simulink model "Quadcopter_model"  (R2022b)
settings: Solver=FixedStepAuto  StartTime=0.0  StopTime=5  FixedStep=Ts  RelTol=1e-3
undefined symbols (not defined in the file or in its folder): Cm, Ct, g, Ir, Ixx, Iyy, Izz, Length, linear_mat_A, linear_mat_B, linear_mat_C, linear_mat_D, mass
settings Model: Creator=Bw Jiang  LastModifiedBy=Bw Jiang

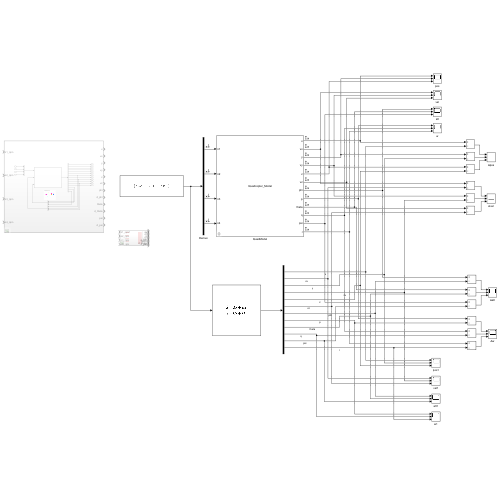
[thumbnail: Simulink's stored preview of the top-level diagram]
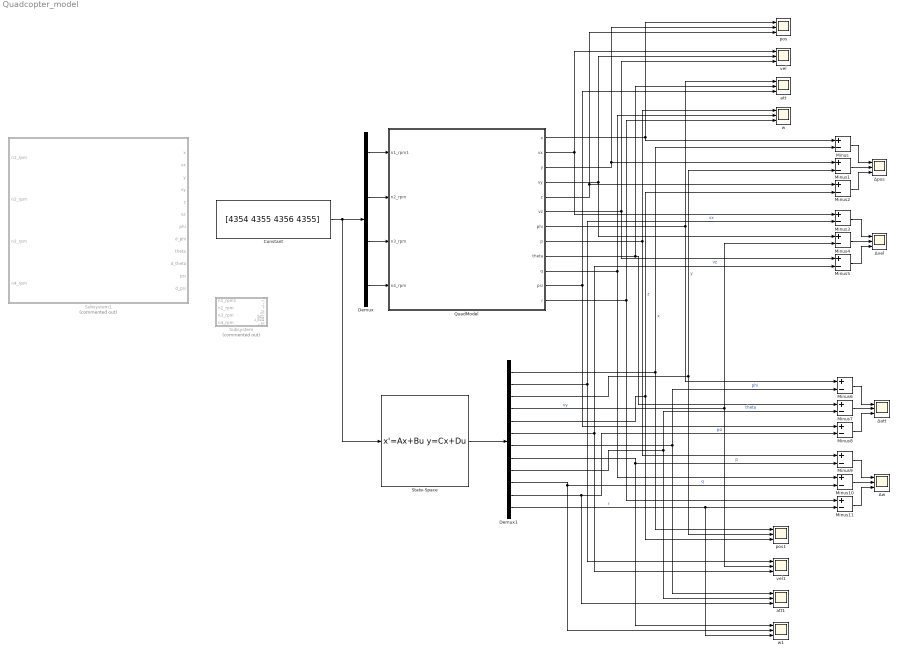
== system Quadcopter_model ==
  Constant : Constant  Value=[4354 4355 4356 4355]
  Demux : Demux
  Demux1 : Demux  Outputs=12
  Minus{,1..11} (12 alike) : Sum  Inputs=+-
  QuadModel : Subsystem  mask{g=g, mass=mass, I_xx=Ixx, I_yy=Iyy, I_zz=Izz, I_r=Ir, L=Length, C_M=Cm, C_T=Ct}
      mask prompts: g "Gravity"; I_xx "Inertia_xx"; I_yy "Inertia_yy"; I_zz "Inertia_zz"; I_r "Inertia_per_rotor"; L "Length"
      mask DialogControl ParameterGroupVar Prompt: 参数
      mask Display:
      | disp('Quadcopter_Model');
      | 
      | port_label('input', 1, 'n1');
      | port_label('input', 2, 'n2');
      | port_label('input', 3, 'n3');
      | port_label('input', 4, 'n4');
      | 
      | port_label('output', 1, 'x');
      | port_label('output', 2, 'vx');
      | port_label('output', 3, 'y');
      | port_label('output', 4, 'vy');
      | port_label('output', 5, 'z');
      | port_label('output', 6, 'vz');
      | port_label('output', 7, 'phi');
      | port_label('output', 8, 'p');
      | port_label('output', 9, 'theta');
      | port_label('output', 10, 'q');
      | port_label('output', 11, 'psi');
      | port_label('output', 12, 'r');
  State-Space : StateSpace  A=linear_mat_A  B=linear_mat_B  C=linear_mat_C  D=linear_mat_D  InitialCondition=0
  Subsystem : Subsystem  Commented=on
  Subsystem1 : Subsystem  Commented=on
  att : Scope  NumInputPorts=3
  att1 : Scope  NumInputPorts=3
  pos : Scope  NumInputPorts=3
  pos1 : Scope  NumInputPorts=3
  vel : Scope  NumInputPorts=3
  vel1 : Scope  NumInputPorts=3
  w : Scope  NumInputPorts=3
  w1 : Scope  NumInputPorts=3
  Δatt : Scope  NumInputPorts=3
  Δpos : Scope  NumInputPorts=3
  Δvel : Scope  NumInputPorts=3
  Δw : Scope  NumInputPorts=3
  wires:
  Demux/1 -> QuadModel/1(n1_rpm1)
  Demux/2 -> QuadModel/2(n2_rpm)
  Demux/3 -> QuadModel/3(n3_rpm)
  Demux/4 -> QuadModel/4(n4_rpm)
  Constant/1 -> Demux/1, State-Space/1
  QuadModel/1(x) -> Minus/1, pos/1
  QuadModel/3(y) -> pos/2, Minus1/1
  QuadModel/5(z) -> pos/3, Minus2/1
  QuadModel/2(vx) -> Minus3/1, vel/1
  QuadModel/4(vy) -> vel/2, Minus4/1
  QuadModel/6(vz) -> Minus5/1, vel/3
  QuadModel/7(phi) -> Minus6/1, att/1
  QuadModel/9(theta) -> Minus7/1, att/2
  QuadModel/11(psi) -> Minus8/1, att/3
  QuadModel/8(p) -> Minus9/1, w/1
  QuadModel/10(q) -> Minus10/1, w/2
  QuadModel/12(r) -> Minus11/1, w/3
  State-Space/1 -> Demux1/1
  Demux1/1 -> Minus/2, pos1/1  "x"
  Demux1/3 -> Minus1/2, pos1/2  "y"
  Demux1/5 -> Minus2/2, pos1/3  "z"
  Demux1/2 -> Minus3/2, vel1/1  "vx"
  Demux1/4 -> Minus4/2, vel1/2  "vy"
  Demux1/6 -> Minus5/2, vel1/3  "vz"
  Demux1/7 -> Minus6/2, att1/1  "phi"
  Demux1/9 -> Minus7/2, att1/2  "theta"
  Demux1/11 -> Minus8/2, att1/3  "psi"
  Demux1/12 -> Minus11/2, w1/3  "r"
  Demux1/10 -> w1/2, Minus10/2  "q"
  Demux1/8 -> w1/1, Minus9/2  "p"
  Minus/1 -> Δpos/1
  Minus1/1 -> Δpos/2
  Minus2/1 -> Δpos/3
  Minus3/1 -> Δvel/1
  Minus5/1 -> Δvel/3
  Minus4/1 -> Δvel/2
  Minus6/1 -> Δatt/1
  Minus7/1 -> Δatt/2
  Minus8/1 -> Δatt/3
  Minus9/1 -> Δw/1
  Minus10/1 -> Δw/2
  Minus11/1 -> Δw/3

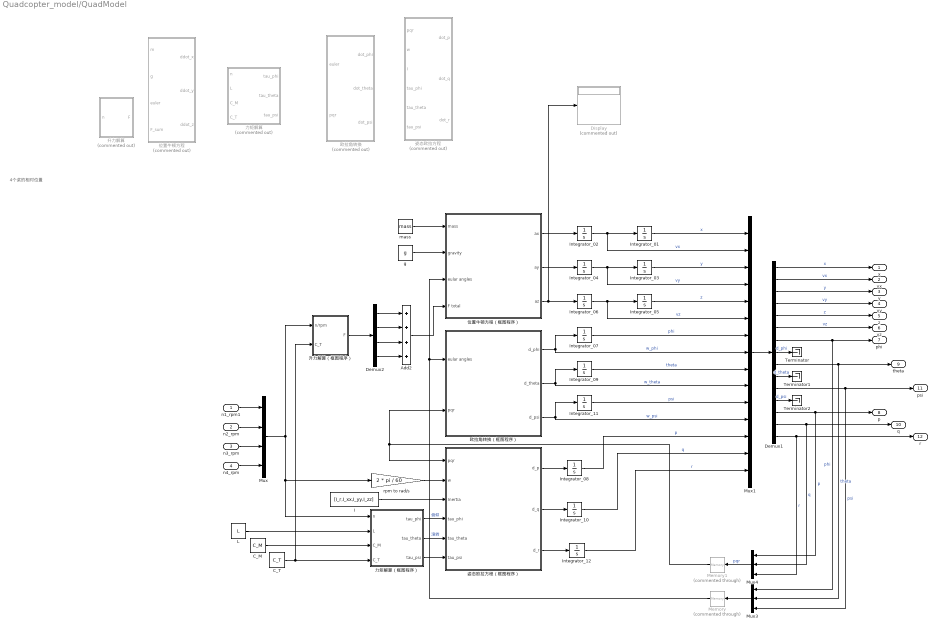
== system Quadcopter_model/QuadModel ==
  note: 4个桨的相对位置
  n1_rpm1 : Inport
  n2_rpm : Inport  Port=2
  n3_rpm : Inport  Port=3
  n4_rpm : Inport  Port=4
  Add2 : Sum  Inputs=++++
  C_M : Constant  Value=C_M
  C_T : Constant  Value=C_T
  Demux1 : Demux  Outputs=15
  Demux2 : Demux
  Display : Display  Commented=on
  I : Constant  Value=[I_r,I_xx,I_yy,I_zz]
  Integrator_01 : Integrator
  Integrator_02 : Integrator
  Integrator_03 : Integrator
  Integrator_04 : Integrator
  Integrator_05 : Integrator
  Integrator_06 : Integrator
  Integrator_07 : Integrator
  Integrator_08 : Integrator
  Integrator_09 : Integrator
  Integrator_10 : Integrator
  Integrator_11 : Integrator
  Integrator_12 : Integrator
  L : Constant  Value=L
  Memory : Memory  Commented=through  InheritSampleTime=on
  Memory1 : Memory  Commented=through  InheritSampleTime=on
  Mux : Mux
  Mux1 : Mux  Inputs=15
  Mux3 : Mux  Inputs=3
  Mux4 : Mux  Inputs=3
  Terminator : Terminator
  Terminator1 : Terminator
  Terminator2 : Terminator
  g : Constant  Value=g
  mass : Constant  Value=mass
  rpm to rad/s : Gain  Gain=2 * pi / 60
  位置牛顿方程 : MATLAB Function  Commented=on  TreatAsAtomicUnit=on
  位置牛顿方程（框图程序） : Subsystem
  力矩解算 : MATLAB Function  Commented=on  TreatAsAtomicUnit=on
  力矩解算（框图程序） : Subsystem
  升力解算 : MATLAB Function  Commented=on  TreatAsAtomicUnit=on
  升力解算（框图程序） : Subsystem
  姿态欧拉方程 : MATLAB Function  Commented=on  TreatAsAtomicUnit=on
  姿态欧拉方程（框图程序） : Subsystem
  欧拉角转换 : MATLAB Function  Commented=on  TreatAsAtomicUnit=on
  欧拉角转换（框图程序） : Subsystem
  x : Outport
  vx : Outport  Port=2
  y : Outport  Port=3
  vy : Outport  Port=4
  z : Outport  Port=5
  vz : Outport  Port=6
  phi : Outport  Port=7
  p : Outport  Port=8
  theta : Outport  Port=9
  q : Outport  Port=10
  psi : Outport  Port=11
  r : Outport  Port=12
  wires:
  Demux1/15 -> r/1, Mux4/3  "r"
  Demux1/13 -> Mux4/1, p/1  "p"
  Mux4/1 -> Memory1/1  "pqr"
  Demux1/9 -> theta/1, Mux3/2  "theta"
  Demux1/1 -> x/1  "x"
  Demux1/2 -> vx/1  "vx"
  Demux1/11 -> psi/1, Mux3/3  "psi"
  Demux1/4 -> vy/1  "vy"
  Demux1/3 -> y/1  "y"
  Demux1/5 -> z/1  "z"
  Mux1/1 -> Demux1/1
  Demux1/6 -> vz/1  "vz"
  Demux1/7 -> phi/1, Mux3/1  "phi"
  Mux3/1 -> Memory/1
  Demux1/14 -> q/1, Mux4/2  "q"
  Demux1/8 -> Terminator/1  "d_phi"
  Demux1/10 -> Terminator1/1  "d_theta"
  Demux1/12 -> Terminator2/1  "d_psi"
  n1_rpm1/1 -> Mux/1
  n2_rpm/1 -> Mux/2
  n4_rpm/1 -> Mux/4
  n3_rpm/1 -> Mux/3
  欧拉角转换（框图程序）/2(d_theta) -> Integrator_09/1, Mux1/10  "w_theta"
  欧拉角转换（框图程序）/3(d_psi) -> Integrator_11/1, Mux1/12  "w_psi"
  欧拉角转换（框图程序）/1(d_phi) -> Integrator_07/1, Mux1/8  "w_phi"
  力矩解算（框图程序）/3(tau_psi) -> 姿态欧拉方程（框图程序）/6(tau_psi)
  力矩解算（框图程序）/2(tau_theta) -> 姿态欧拉方程（框图程序）/5(tau_theta)  "滚转"
  姿态欧拉方程（框图程序）/2(d_q) -> Integrator_10/1
  姿态欧拉方程（框图程序）/3(d_r) -> Integrator_12/1
  mass/1 -> 位置牛顿方程（框图程序）/1(mass)
  Add2/1 -> 位置牛顿方程（框图程序）/4(F total)
  g/1 -> 位置牛顿方程（框图程序）/2(gravity)
  位置牛顿方程（框图程序）/3(az) -> Display/1, Integrator_06/1
  位置牛顿方程（框图程序）/2(ay) -> Integrator_04/1
  Integrator_09/1 -> Mux1/9  "theta"
  力矩解算（框图程序）/1(tau_phi) -> 姿态欧拉方程（框图程序）/4(tau_phi)  "俯仰"
  Integrator_02/1 -> Integrator_01/1, Mux1/2  "vx"
  Integrator_03/1 -> Mux1/3  "y"
  Demux2/3 -> Add2/3
  Integrator_12/1 -> Mux1/15  "r"
  rpm to rad/s/1 -> 姿态欧拉方程（框图程序）/2(w)
  Integrator_11/1 -> Mux1/11  "psi"
  Integrator_04/1 -> Mux1/4, Integrator_03/1  "vy"
  Mux/1 -> 力矩解算（框图程序）/1(n), rpm to rad/s/1, 升力解算（框图程序）/1(n/rpm)
  Memory1/1 -> 欧拉角转换（框图程序）/2(pqr), 姿态欧拉方程（框图程序）/1(pqr)
  位置牛顿方程（框图程序）/1(ax) -> Integrator_02/1
  Demux2/1 -> Add2/1
  Integrator_01/1 -> Mux1/1  "x"
  Integrator_10/1 -> Mux1/14  "q"
  姿态欧拉方程（框图程序）/1(d_p) -> Integrator_08/1
  Integrator_07/1 -> Mux1/7  "phi"
  Demux2/2 -> Add2/2
  L/1 -> 力矩解算（框图程序）/2(L)
  I/1 -> 姿态欧拉方程（框图程序）/3(Inertia)
  C_M/1 -> 力矩解算（框图程序）/3(C_M)
  升力解算（框图程序）/1(F) -> Demux2/1
  C_T/1 -> 升力解算（框图程序）/2(C_T), 力矩解算（框图程序）/4(C_T)
  Integrator_05/1 -> Mux1/5  "z"
  Demux2/4 -> Add2/4
  Integrator_06/1 -> Mux1/6, Integrator_05/1  "vz"
  Integrator_08/1 -> Mux1/13  "p"
  Memory/1 -> 位置牛顿方程（框图程序）/3(eular angles), 欧拉角转换（框图程序）/1(eular angles)

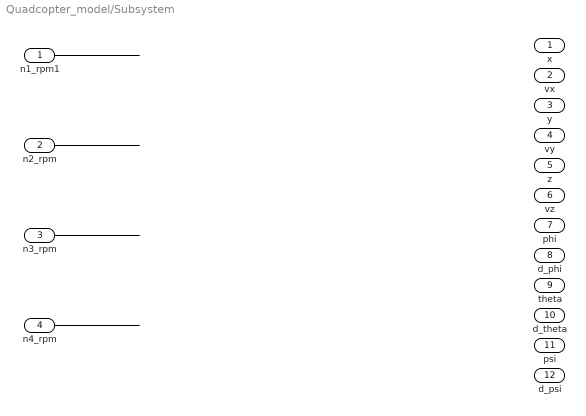
== system Quadcopter_model/Subsystem ==
  n1_rpm1 : Inport
  n2_rpm : Inport  Port=2
  n3_rpm : Inport  Port=3
  n4_rpm : Inport  Port=4
  x : Outport
  vx : Outport  Port=2
  y : Outport  Port=3
  vy : Outport  Port=4
  z : Outport  Port=5
  vz : Outport  Port=6
  phi : Outport  Port=7
  d_phi : Outport  Port=8
  theta : Outport  Port=9
  d_theta : Outport  Port=10
  psi : Outport  Port=11
  d_psi : Outport  Port=12
  wires:
  n2_rpm/1 -> ?
  n3_rpm/1 -> ?
  n4_rpm/1 -> ?
  n1_rpm1/1 -> ?
  ? -> theta/1
  ? -> x/1
  ? -> d_psi/1
  ? -> vx/1
  ? -> y/1
  ? -> vy/1
  ? -> psi/1
  ? -> d_phi/1
  ? -> vz/1
  ? -> d_theta/1
  ? -> z/1
  ? -> phi/1

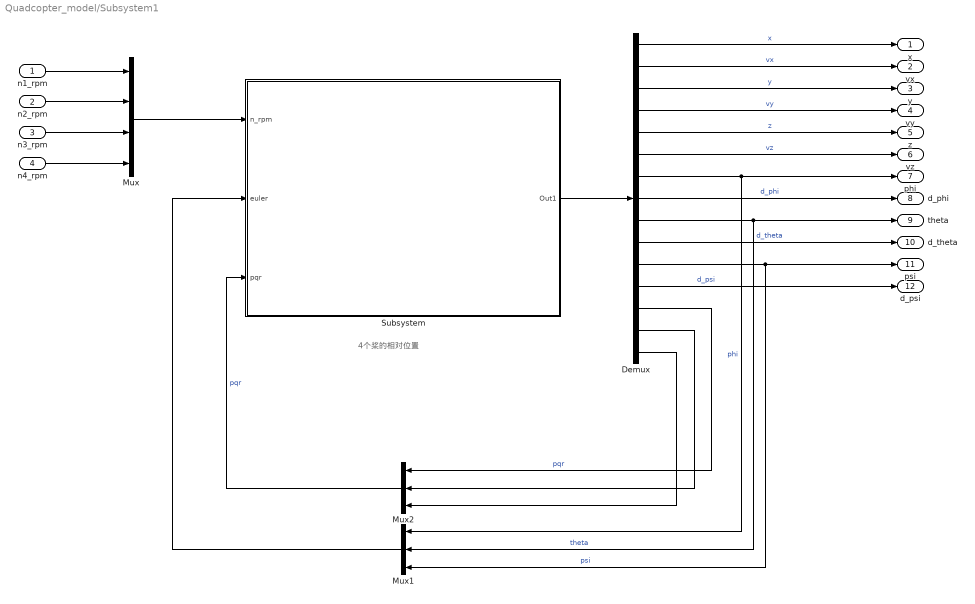
== system Quadcopter_model/Subsystem1 ==
  note: 4个桨的相对位置
  n1_rpm : Inport
  n2_rpm : Inport  Port=2
  n3_rpm : Inport  Port=3
  n4_rpm : Inport  Port=4
  Demux : Demux  Outputs=15
  Mux : Mux
  Mux1 : Mux  Inputs=3
  Mux2 : Mux  Inputs=3
  Subsystem : Subsystem
  x : Outport
  vx : Outport  Port=2
  y : Outport  Port=3
  vy : Outport  Port=4
  z : Outport  Port=5
  vz : Outport  Port=6
  phi : Outport  Port=7
  d_phi : Outport  Port=8
  theta : Outport  Port=9
  d_theta : Outport  Port=10
  psi : Outport  Port=11
  d_psi : Outport  Port=12
  wires:
  Demux/11 -> psi/1, Mux1/3  "psi"
  Demux/14 -> Mux2/2
  Mux2/1 -> Subsystem/3(pqr)  "pqr"
  Demux/13 -> Mux2/1  "pqr"
  Subsystem/1(Out1) -> Demux/1
  Demux/9 -> theta/1, Mux1/2  "theta"
  Demux/15 -> Mux2/3
  Demux/7 -> phi/1, Mux1/1  "phi"
  Demux/5 -> z/1  "z"
  Mux1/1 -> Subsystem/2(euler)
  Demux/8 -> d_phi/1  "d_phi"
  Demux/2 -> vx/1  "vx"
  n1_rpm/1 -> Mux/1
  Demux/12 -> d_psi/1  "d_psi"
  Demux/10 -> d_theta/1  "d_theta"
  Demux/4 -> vy/1  "vy"
  Demux/6 -> vz/1  "vz"
  Demux/3 -> y/1  "y"
  Demux/1 -> x/1  "x"
  n3_rpm/1 -> Mux/3
  n4_rpm/1 -> Mux/4
  n2_rpm/1 -> Mux/2
  Mux/1 -> Subsystem/1(n_rpm)

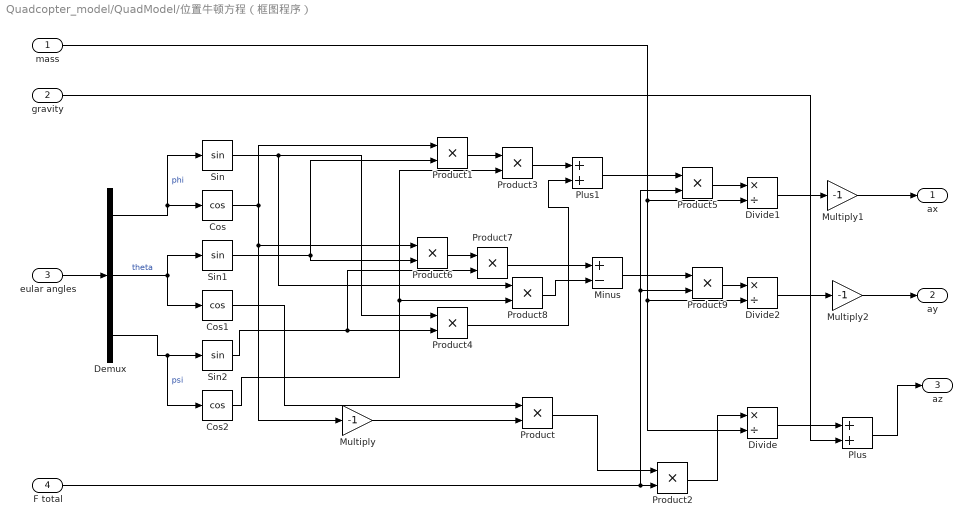
== system Quadcopter_model/QuadModel/位置牛顿方程（框图程序） ==
  mass : Inport
  gravity : Inport  Port=2
  eular angles : Inport  Port=3
  F total : Inport  Port=4
  Cos : Trigonometry  Operator=cos
  Cos1 : Trigonometry  Operator=cos
  Cos2 : Trigonometry  Operator=cos
  Demux : Demux  Outputs=3
  Divide : Product  Inputs=*/
  Divide1 : Product  Inputs=*/
  Divide2 : Product  Inputs=*/
  Minus : Sum  Inputs=+-
  Multiply : Gain  Gain=-1
  Multiply1 : Gain  Gain=-1
  Multiply2 : Gain  Gain=-1
  Plus : Sum
  Plus1 : Sum
  Product{,1..9} (10 alike) : Product
  Sin : Trigonometry
  Sin1 : Trigonometry
  Sin2 : Trigonometry
  ax : Outport
  ay : Outport  Port=2
  az : Outport  Port=3
  wires:
  eular angles/1 -> Demux/1
  Demux/1 -> Sin/1, Cos/1  "phi"
  Demux/2 -> Sin1/1, Cos1/1  "theta"
  Demux/3 -> Cos2/1, Sin2/1  "psi"
  Cos/1 -> Product6/1, Multiply/1, Product1/1
  Multiply/1 -> Product/2
  Cos1/1 -> Product/1
  F total/1 -> Product5/2, Product9/2, Product2/2
  Product/1 -> Product2/1
  Product2/1 -> Divide/1
  mass/1 -> Divide2/2, Divide/2, Divide1/2
  Divide/1 -> Plus/1
  gravity/1 -> Plus/2
  Plus/1 -> az/1
  Sin1/1 -> Product1/2, Product6/2
  Product1/1 -> Product3/1
  Cos2/1 -> Product8/2, Product3/2
  Product3/1 -> Plus1/1
  Sin/1 -> Product8/1, Product4/1
  Sin2/1 -> Product7/2, Product4/2
  Product4/1 -> Plus1/2
  Plus1/1 -> Product5/1
  Product5/1 -> Divide1/1
  Divide1/1 -> Multiply1/1
  Multiply1/1 -> ax/1
  Product6/1 -> Product7/1
  Product7/1 -> Minus/1
  Product8/1 -> Minus/2
  Minus/1 -> Product9/1
  Product9/1 -> Divide2/1
  Multiply2/1 -> ay/1
  Divide2/1 -> Multiply2/1

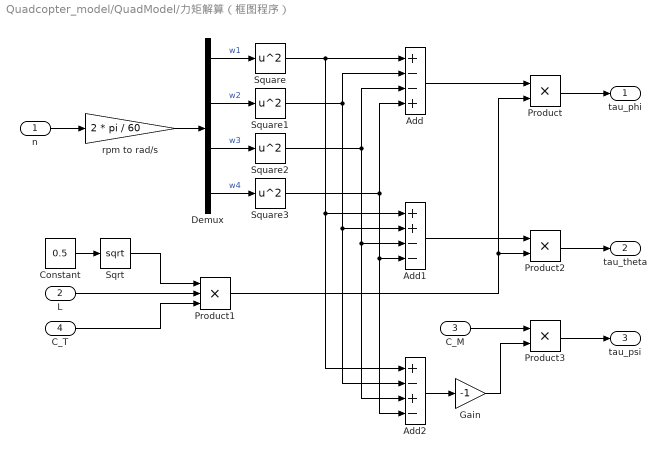
== system Quadcopter_model/QuadModel/力矩解算（框图程序） ==
  n : Inport
  L : Inport  Port=2
  C_M : Inport  Port=3
  C_T : Inport  Port=4
  Add : Sum  Inputs=+--+
  Add1 : Sum  Inputs=++--
  Add2 : Sum  Inputs=+-+-
  Constant : Constant  Value=0.5
  Demux : Demux
  Gain : Gain  Gain=-1
  Product : Product
  Product1 : Product  Inputs=3
  Product2 : Product
  Product3 : Product
  Sqrt : Sqrt
  Square{,1..3} (4 alike) : Math  Operator=square
  rpm to rad/s : Gain  Gain=2 * pi / 60
  tau_phi : Outport
  tau_theta : Outport  Port=2
  tau_psi : Outport  Port=3
  wires:
  rpm to rad/s/1 -> Demux/1
  n/1 -> rpm to rad/s/1
  Demux/1 -> Square/1  "w1"
  Demux/2 -> Square1/1  "w2"
  Demux/3 -> Square2/1  "w3"
  Demux/4 -> Square3/1  "w4"
  Square/1 -> Add1/1, Add2/1, Add/1
  Square1/1 -> Add1/2, Add2/2, Add/2
  Square2/1 -> Add2/3, Add1/3, Add/3
  Square3/1 -> Add2/4, Add1/4, Add/4
  Add/1 -> Product/1
  L/1 -> Product1/2
  C_T/1 -> Product1/3
  Constant/1 -> Sqrt/1
  Sqrt/1 -> Product1/1
  Product1/1 -> Product/2, Product2/2
  Product/1 -> tau_phi/1
  Add1/1 -> Product2/1
  Product2/1 -> tau_theta/1
  Add2/1 -> Gain/1
  C_M/1 -> Product3/1
  Product3/1 -> tau_psi/1
  Gain/1 -> Product3/2

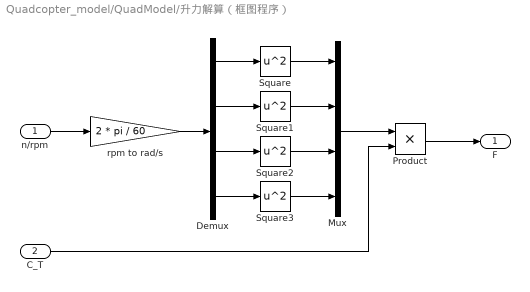
== system Quadcopter_model/QuadModel/升力解算（框图程序） ==
  n/rpm : Inport
  C_T : Inport  Port=2
  Demux : Demux
  Mux : Mux
  Product : Product
  Square{,1..3} (4 alike) : Math  Operator=square
  rpm to rad/s : Gain  Gain=2 * pi / 60
  F : Outport
  wires:
  n/rpm/1 -> rpm to rad/s/1
  rpm to rad/s/1 -> Demux/1
  Demux/1 -> Square/1
  Demux/2 -> Square1/1
  Demux/3 -> Square2/1
  Demux/4 -> Square3/1
  Square3/1 -> Mux/4
  Square2/1 -> Mux/3
  Square1/1 -> Mux/2
  Square/1 -> Mux/1
  Mux/1 -> Product/1
  C_T/1 -> Product/2
  Product/1 -> F/1

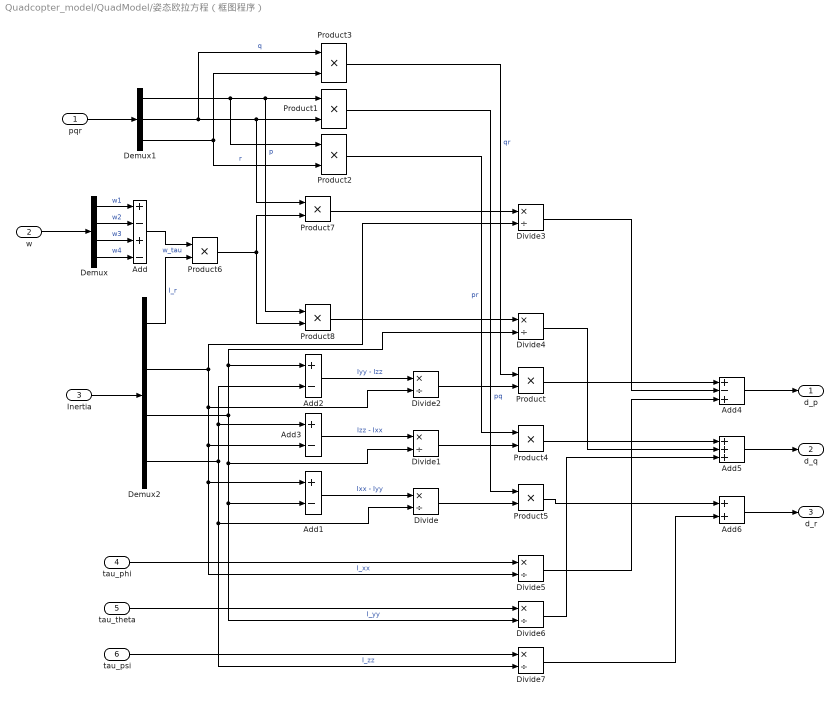
== system Quadcopter_model/QuadModel/姿态欧拉方程（框图程序） ==
  pqr : Inport
  w : Inport  Port=2
  Inertia : Inport  Port=3
  tau_phi : Inport  Port=4
  tau_theta : Inport  Port=5
  tau_psi : Inport  Port=6
  Add : Sum  Inputs=+-+-
  Add1 : Sum  Inputs=+-
  Add2 : Sum  Inputs=+-
  Add3 : Sum  Inputs=+-
  Add4 : Sum  Inputs=+-+
  Add5 : Sum  Inputs=+++
  Add6 : Sum
  Demux : Demux
  Demux1 : Demux  Outputs=3
  Demux2 : Demux
  Divide{,1..7} (8 alike) : Product  Inputs=*/
  Product{,1..8} (9 alike) : Product
  d_p : Outport
  d_q : Outport  Port=2
  d_r : Outport  Port=3
  wires:
  w/1 -> Demux/1
  pqr/1 -> Demux1/1
  Inertia/1 -> Demux2/1
  Demux/1 -> Add/1  "w1"
  Demux/2 -> Add/2  "w2"
  Demux/3 -> Add/3  "w3"
  Demux/4 -> Add/4  "w4"
  Demux2/2 -> Add3/2, Add1/1, Divide5/2, Divide2/2, Divide3/2  "I_xx"
  Demux2/3 -> Divide4/2, Add2/1, Divide1/2, Divide6/2, Add1/2  "I_yy"
  Demux2/4 -> Add2/2, Add3/1, Divide7/2, Divide/2  "I_zz"
  Add1/1 -> Divide/1  "Ixx - Iyy"
  Add3/1 -> Divide1/1  "Izz - Ixx"
  Add2/1 -> Divide2/1  "Iyy - Izz"
  Divide2/1 -> Product/2
  Demux1/2 -> Product3/1, Product1/2, Product7/1  "q"
  Demux1/1 -> Product2/1, Product1/1, Product8/1  "p"
  Demux1/3 -> Product2/2, Product3/2  "r"
  Divide/1 -> Product5/2
  Divide1/1 -> Product4/2
  Product3/1 -> Product/1  "qr"
  Product1/1 -> Product5/1  "pq"
  Product2/1 -> Product4/1  "pr"
  Add/1 -> Product6/1  "w_tau"
  Demux2/1 -> Product6/2  "I_r"
  Product6/1 -> Product8/2, Product7/2
  Product7/1 -> Divide3/1
  Product8/1 -> Divide4/1
  tau_phi/1 -> Divide5/1
  tau_theta/1 -> Divide6/1
  tau_psi/1 -> Divide7/1
  Product/1 -> Add4/1
  Divide3/1 -> Add4/2
  Divide5/1 -> Add4/3
  Product4/1 -> Add5/1
  Divide4/1 -> Add5/2
  Divide6/1 -> Add5/3
  Add4/1 -> d_p/1
  Add5/1 -> d_q/1
  Product5/1 -> Add6/1
  Divide7/1 -> Add6/2
  Add6/1 -> d_r/1

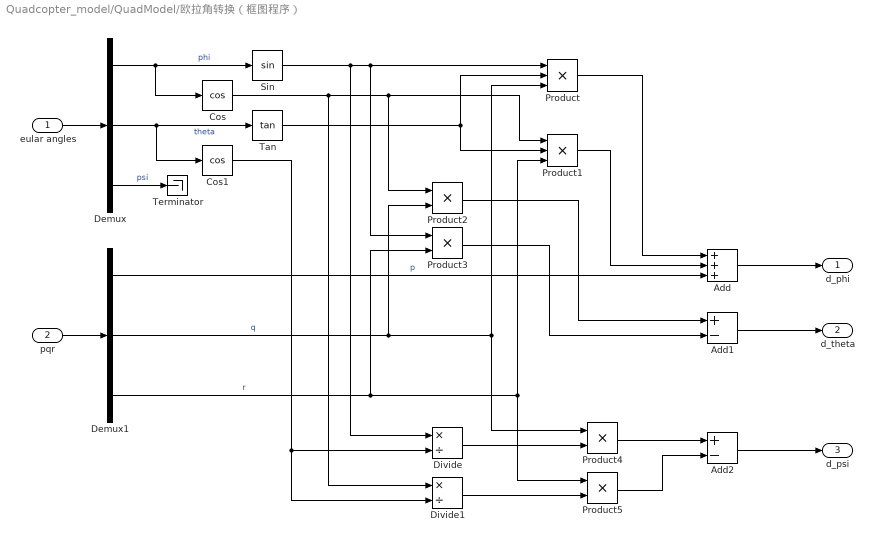
== system Quadcopter_model/QuadModel/欧拉角转换（框图程序） ==
  eular angles : Inport
  pqr : Inport  Port=2
  Add : Sum  Inputs=+++
  Add1 : Sum  Inputs=+-
  Add2 : Sum  Inputs=+-
  Cos : Trigonometry  Operator=cos
  Cos1 : Trigonometry  Operator=cos
  Demux : Demux  Outputs=3
  Demux1 : Demux  Outputs=3
  Divide : Product  Inputs=*/
  Divide1 : Product  Inputs=*/
  Product : Product  Inputs=3
  Product1 : Product  Inputs=3
  Product{2..5} (4 alike) : Product
  Sin : Trigonometry
  Tan : Trigonometry  Operator=tan
  Terminator : Terminator
  d_phi : Outport
  d_theta : Outport  Port=2
  d_psi : Outport  Port=3
  wires:
  eular angles/1 -> Demux/1
  pqr/1 -> Demux1/1
  Demux1/1 -> Add/3  "p"
  Add/1 -> d_phi/1
  Add1/1 -> d_theta/1
  Add2/1 -> d_psi/1
  Demux/1 -> Sin/1, Cos/1  "phi"
  Demux/2 -> Cos1/1, Tan/1  "theta"
  Demux/3 -> Terminator/1  "psi"
  Demux1/2 -> Product2/2, Product4/1, Product/3  "q"
  Sin/1 -> Divide/1, Product3/1, Product/1
  Tan/1 -> Product1/2, Product/2
  Cos/1 -> Divide1/1, Product2/1, Product1/1
  Demux1/3 -> Product3/2, Product1/3, Product5/1  "r"
  Product/1 -> Add/1
  Product1/1 -> Add/2
  Product2/1 -> Add1/1
  Product3/1 -> Add1/2
  Cos1/1 -> Divide1/2, Divide/2
  Divide/1 -> Product4/2
  Product4/1 -> Add2/1
  Divide1/1 -> Product5/2
  Product5/1 -> Add2/2

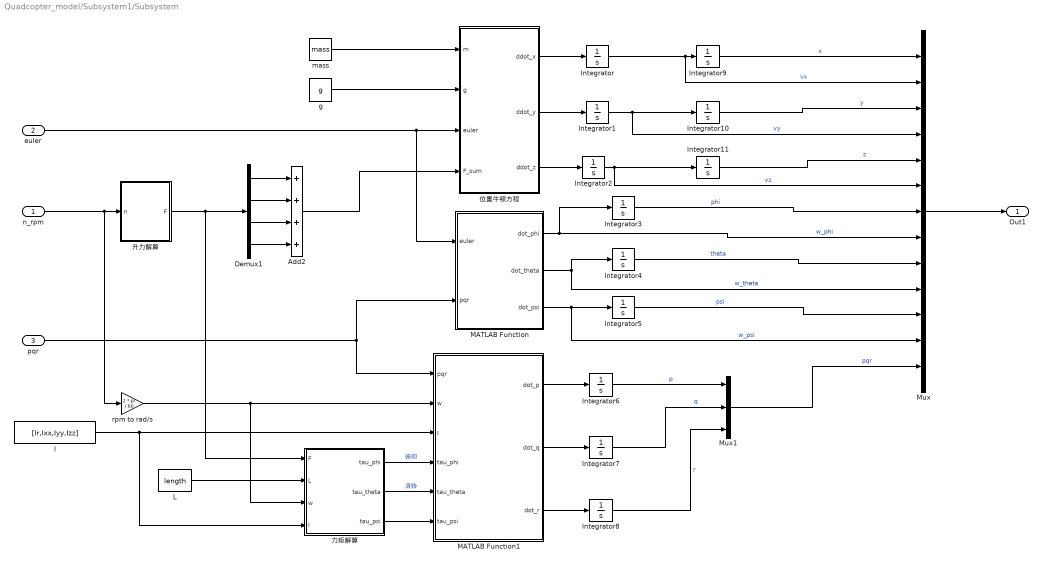
== system Quadcopter_model/Subsystem1/Subsystem ==
  n_rpm : Inport  PortDimensions=4
  euler : Inport  Port=2  PortDimensions=3
  pqr : Inport  Port=3  PortDimensions=3
  Add2 : Sum  Inputs=++++
  Demux1 : Demux
  I : Constant  Value=[Ir,Ixx,Iyy,Izz]
  Integrator{,1..11} (12 alike) : Integrator
  L : Constant  Value=length
  MATLAB Function : MATLAB Function  TreatAsAtomicUnit=on
  MATLAB Function1 : MATLAB Function  TreatAsAtomicUnit=on
  Mux : Mux  Inputs=13
  Mux1 : Mux  Inputs=3
  g : Constant  Value=g
  mass : Constant  Value=mass
  rpm to rad/s : Gain  Gain=2 * pi / 60
  位置牛顿方程 : MATLAB Function  TreatAsAtomicUnit=on
  力矩解算 : MATLAB Function  TreatAsAtomicUnit=on
  升力解算 : MATLAB Function  TreatAsAtomicUnit=on
  Out1 : Outport
  wires:
  MATLAB Function1/1(dot_p) -> Integrator6/1
  Demux1/4 -> Add2/4
  pqr/1 -> MATLAB Function/2(pqr), MATLAB Function1/1(pqr)
  位置牛顿方程/2(ddot_y) -> Integrator1/1
  MATLAB Function1/2(dot_q) -> Integrator7/1
  n_rpm/1 -> 升力解算/1(n), rpm to rad/s/1
  I/1 -> 力矩解算/4(I), MATLAB Function1/3(I)
  位置牛顿方程/3(ddot_z) -> Integrator2/1
  Mux/1 -> Out1/1
  g/1 -> 位置牛顿方程/2(g)
  位置牛顿方程/1(ddot_x) -> Integrator/1
  Integrator7/1 -> Mux1/2  "q"
  Demux1/1 -> Add2/1
  力矩解算/1(tau_phi) -> MATLAB Function1/4(tau_phi)  "俯仰"
  Integrator6/1 -> Mux1/1  "p"
  euler/1 -> MATLAB Function/1(euler), 位置牛顿方程/3(euler)
  Integrator10/1 -> Mux/3  "y"
  Integrator4/1 -> Mux/9  "theta"
  力矩解算/3(tau_psi) -> MATLAB Function1/6(tau_psi)
  Demux1/2 -> Add2/2
  Add2/1 -> 位置牛顿方程/4(F_sum)
  Integrator8/1 -> Mux1/3  "r"
  mass/1 -> 位置牛顿方程/1(m)
  力矩解算/2(tau_theta) -> MATLAB Function1/5(tau_theta)  "滚转"
  Demux1/3 -> Add2/3
  Integrator11/1 -> Mux/5  "z"
  Integrator9/1 -> Mux/1  "x"
  Integrator/1 -> Mux/2, Integrator9/1  "vx"
  Integrator3/1 -> Mux/7  "phi"
  Integrator1/1 -> Mux/4, Integrator10/1  "vy"
  Integrator2/1 -> Integrator11/1, Mux/6  "vz"
  Integrator5/1 -> Mux/11  "psi"
  MATLAB Function1/3(dot_r) -> Integrator8/1
  MATLAB Function/3(dot_psi) -> Mux/12, Integrator5/1  "w_psi"
  MATLAB Function/2(dot_theta) -> Mux/10, Integrator4/1  "w_theta"
  MATLAB Function/1(dot_phi) -> Integrator3/1, Mux/8  "w_phi"
  Mux1/1 -> Mux/13  "pqr"
  升力解算/1(F) -> 力矩解算/1(F), Demux1/1
  L/1 -> 力矩解算/2(L)
  rpm to rad/s/1 -> 力矩解算/3(w), MATLAB Function1/2(w)

== matlab function Quadcopter_model/QuadModel/升力解算 ==
  data: n input; F output
function F = fcn(n)
%% Input Vars
% n - rpm

%% Output Vars
% F - N

%% Mid Vars
% omega - rad/s

%% Code

% F = n .* n * 2.414e-7 * 2;

omega = n / 60 * 2 * pi;
F = omega .* omega * 1.11e-5;

end

== matlab function Quadcopter_model/QuadModel/姿态欧拉方程 ==
  data: pqr input; dot_p output; w input; I input; dot_q output; dot_r output; tau_phi input; tau_theta input; tau_psi input
function [dot_p, dot_q, dot_r] = fcn(pqr, w, I, tau_phi, tau_theta, tau_psi)

w1 = w(1);
w2 = w(2);
w3 = w(3);
w4 = w(4);

p = pqr(1);
q = pqr(2);
r = pqr(3);

I_r = I(1);
I_xx = I(2);
I_yy = I(3);
I_zz = I(4);

w_tau = w1 - w2 + w3 - w4;

dot_p = (I_yy - I_zz) / I_xx * q * r - I_r * q / I_xx * w_tau + tau_phi / I_xx;
dot_q = (I_zz - I_xx) / I_yy * p * r + I_r * p / I_yy * w_tau + tau_theta / I_yy;
dot_r = (I_xx - I_yy) / I_zz * q * p + tau_psi / I_zz;

end

== matlab function Quadcopter_model/Subsystem1/Subsystem/MATLAB Function ==
  data: euler input; pqr input; dot_phi output; dot_theta output; dot_psi output
function [dot_phi, dot_theta, dot_psi] = fcn(euler, pqr)

% 角加速度的坐标转换，从机体系b到惯性系e

p = pqr(1);
q = pqr(2);
r = pqr(3);

phi =euler(1);
theta = euler(2);
psi = euler(3);

mat = [
    1, tan(theta) * sin(phi), tan(theta) * cos(phi);
    0, cos(phi), -sin(phi);
    0, sin(phi) / cos(theta), cos(phi) / cos(theta)
    ];
body = [p; q; r];
earth = mat * body;

dot_phi = earth(1);
dot_theta = earth(2);
dot_psi = earth(3);

== matlab function Quadcopter_model/Subsystem1/Subsystem/位置牛顿方程 ==
  data: m input; g input; euler input; ddot_x output; F_sum input; ddot_y output; ddot_z output
function [ddot_x, ddot_y, ddot_z] = fcn(m, g, euler, F_sum)

% F_sum恒正

phi =euler(1);
theta = euler(2);
psi = euler(3);

ddot_x = -(cos(phi) * sin(theta) * cos(psi) + sin(phi) * sin(psi)) * F_sum / m;
ddot_y = -(cos(phi) * sin(theta) * sin(psi) - sin(phi) * cos(psi)) * F_sum / m;
ddot_z = -cos(phi) * cos(theta) * F_sum / m + g;

end

== matlab function Quadcopter_model/Subsystem1/Subsystem/MATLAB Function1 ==
  data: pqr input; dot_p output; w input; I input; dot_q output; dot_r output; tau_phi input; tau_theta input; tau_psi input
function [dot_p, dot_q, dot_r] = fcn(pqr, w, I, tau_phi, tau_theta, tau_psi)

w1 = w(1);
w2 = w(2);
w3 = w(3);
w4 = w(4);

p = pqr(1);
q = pqr(2);
r = pqr(3);

I_r = I(1);
I_xx = I(2);
I_yy = I(3);
I_zz = I(4);

w_tau = w1 - w2 + w3 - w4;

dot_p = (I_yy - I_zz) / I_xx * q * r - I_r * q / I_xx * w_tau + tau_phi / I_xx;
dot_q = (I_zz - I_xx) / I_yy * p * r + I_r * p / I_yy * w_tau + tau_theta / I_yy;
dot_r = (I_xx - I_yy) / I_zz * q * p +tau_psi / I_zz;

end

== matlab function Quadcopter_model/Subsystem1/Subsystem/升力解算 ==
  data: n input; F output
function F = fcn(n)

F = n .* n * 2.414e-7 * 2;

end

== matlab function Quadcopter_model/QuadModel/欧拉角转换 ==
  data: euler input; pqr input; dot_phi output; dot_theta output; dot_psi output
function [dot_phi, dot_theta, dot_psi] = fcn(euler, pqr)

% 角加速度的坐标转换，从机体系b到惯性系e

p = pqr(1);
q = pqr(2);
r = pqr(3);

phi =euler(1);
theta = euler(2);
psi = euler(3);

mat = [
    1, tan(theta) * sin(phi), tan(theta) * cos(phi);
    0, cos(phi), -sin(phi);
    0, sin(phi) / cos(theta), cos(phi) / cos(theta)
    ];
body = [p; q; r];
earth = mat * body;

dot_phi = earth(1);
dot_theta = earth(2);
dot_psi = earth(3);

end

== matlab function Quadcopter_model/Subsystem1/Subsystem/力矩解算 ==
  data: F input; tau_phi output; L input; tau_theta output; tau_psi output; w input; I input
function [tau_phi, tau_theta, tau_psi]= fcn(F, L, w, I)

F1=F(1);
F2=F(2);
F3=F(3);
F4=F(4);

w1 = w(1);
w2 = w(2);
w3 = w(3);
w4 = w(4);

I_r = I(1);

w_tau = w1 + w3 - w2 - w4;

tau_phi = (F1+F2-F3-F4) * L;
tau_theta = (F1-F2-F3+F4) * L;
tau_psi = w_tau * I_r;

end

== matlab function Quadcopter_model/QuadModel/位置牛顿方程 ==
  data: m input; g input; euler input; ddot_x output; F_sum input; ddot_y output; ddot_z output
function [ddot_x, ddot_y, ddot_z] = fcn(m, g, euler, F_sum)

% F_sum恒正

phi = euler(1);
theta = euler(2);
psi = euler(3);

ddot_x = -(cos(phi) * sin(theta) * cos(psi) + sin(phi) * sin(psi)) * F_sum / m;
ddot_y = -(cos(phi) * sin(theta) * sin(psi) - sin(phi) * cos(psi)) * F_sum / m;
ddot_z = -cos(phi) * cos(theta) * F_sum / m + g;

end

== matlab function Quadcopter_model/QuadModel/力矩解算 ==
  data: n input; L input; tau_phi output; tau_theta output; tau_psi output; C_M input; C_T input
function [tau_phi, tau_theta, tau_psi]= fcn(n, L, C_M, C_T)
%% Input Vars
% n - rpm
% L - m
% C_M - N*m*s^2/rad^2
% C_T - N*s^2/rad^2

%% Output Vars
% tau - N*m

%% Mid Vars
% w - rad/s

%% Code

% C_T = 1.1e-5;
% C_M = 1.0144e-7;

% F1 = F(1);
% F2 = F(2);
% F3 = F(3);
% F4 = F(4);

w1 = n(1) / 60 * 2 * pi;
w2 = n(2) / 60 * 2 * pi;
w3 = n(3) / 60 * 2 * pi;
w4 = n(4) / 60 * 2 * pi;

% I_r = I(1);

% w_tau = w1 + w3 - w2 - w4;

% 横滚
tau_phi = sqrt(2) / 2 * C_T * L * (w1^2 - w2^2 - w3^2 + w4^2); % tau_phi = (F1+F2-F3-F4) * L;
% 俯仰
tau_theta = sqrt(2) / 2 * C_T * L * (w1^2 + w2^2 - w3^2 - w4^2); % tau_theta = (F1-F2-F3+F4) * L;
% 偏航
tau_psi = C_M * (w1^2 - w2^2 + w3^2 - w4^2); % tau_psi = w_tau * I_r;

end
